simulink model "h"  (R2020a)
settings: Solver=FixedStepAuto  StartTime=0.0  StopTime=10.0  FixedStep=1e-3  RelTol=1e-3  EnableMultiTasking=on
undefined symbols (not defined in the file): D10, D11, D2, D4, D5, D6, D8, PTA0, PTA2, PTB23, PTB9, PTC2, PTD0, PTD2
libraries: frdmk64flib x7
settings Model: ExtModeTrigDuration=5  Creator=qasim  LastModifiedBy=hinda
settings OptimizationCC: EnhancedBackFolding=on  PassReuseOutputArgsAs=Individual arguments  ZeroExternalMemoryAtStartup=off  ZeroInternalMemoryAtStartup=off  MaxStackSize=64  OptimizeBlockOrder=speed  DifferentSizesBufferReuse=on  OptimizationCustomize=off  EfficientTunableParamExpr=on
settings DebuggingCC: ParameterTunabilityLossMsg=error
settings HardwareCC: ProdBitPerPointer=32  ProdBitPerSizeT=32  ProdBitPerPtrDiffT=32  ProdLargestAtomicInteger=Long  ProdLargestAtomicFloat=Double  ProdWordSize=32  ProdHWDeviceType=ARM Compatible->ARM Cortex
settings SFSimCC: MATLABDynamicMemAlloc=off
settings RTWCC: SystemTargetFile=ert.tlc  HardwareBoard=NXP FRDM-K64F  TemplateMakefile=ert_default_tmf  Toolchain=GNU Tools for ARM Embedded Processors
settings CodeAppCC: ForceParamTrailComments=on  IgnoreCustomStorageClasses=off  OperatorAnnotations=on  SimulinkDataObjDesc=on  SFDataObjDesc=on  InsertBlockDesc=on

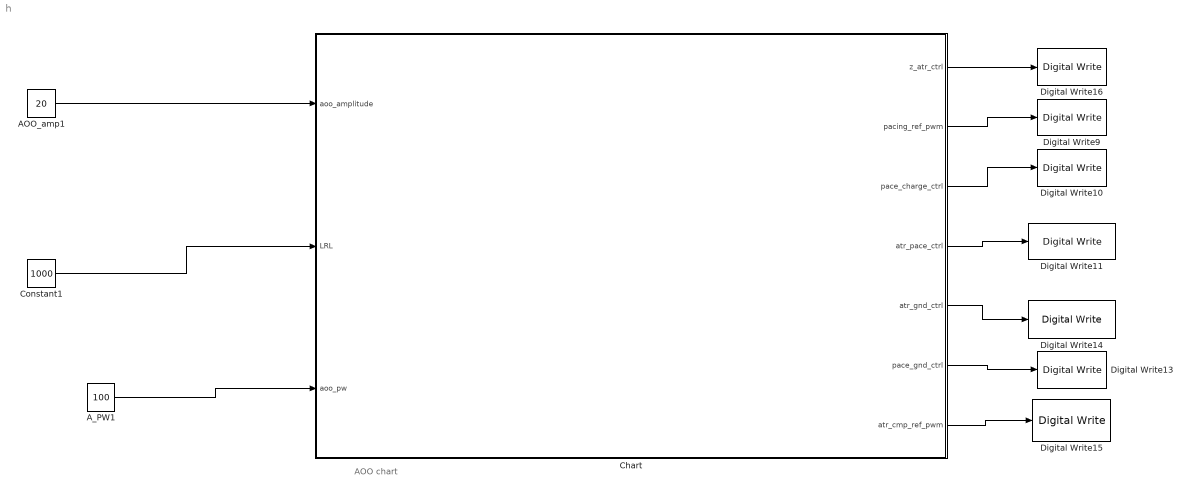
== system h ==
  note: AOO chart
  AOO_amp1 : Constant  Value=20
  A_PW1 : Constant  Value=100
  Chart : Stateflow chart  TreatAsAtomicUnit=on
  Constant1 : Constant  Value=1000
  Digital Write10 : frdmk64flib/Digital Write  Whichpin=PTB9 (D2)
  Digital Write11 : frdmk64flib/Digital Write  Whichpin=PTA0 (D8)
  Digital Write13 : frdmk64flib/Digital Write  Whichpin=PTD0 (D10)
  Digital Write14 : frdmk64flib/Digital Write  Whichpin=PTD2 (D11)
  Digital Write15 : frdmk64flib/Digital Write  Whichpin=PTC2 (D6)
  Digital Write16 : frdmk64flib/Digital Write  Whichpin=PTB23 (D4)
  Digital Write9 : frdmk64flib/Digital Write  Whichpin=PTA2 (D5)
  wires:
  Chart/7(atr_cmp_ref_pwm) -> Digital Write15/1
  Chart/6(pace_gnd_ctrl) -> Digital Write13/1
  Chart/5(atr_gnd_ctrl) -> Digital Write14/1
  Chart/4(atr_pace_ctrl) -> Digital Write11/1
  Chart/3(pace_charge_ctrl) -> Digital Write10/1
  Chart/2(pacing_ref_pwm) -> Digital Write9/1
  Chart/1(z_atr_ctrl) -> Digital Write16/1
  AOO_amp1/1 -> Chart/1(aoo_amplitude)
  Constant1/1 -> Chart/2(LRL)
  A_PW1/1 -> Chart/3(aoo_pw)

== stateflow chart h/Chart ==
  state charging
    entry:
    %charging C22
    %discharging C21
    atr_pace_ctrl = 0; %do not want c22 to discharge
    pacing_ref_pwm = aoo_amplitude; %send in signal
    pace_charge_ctrl = 1;
    pace_gnd_ctrl = 0; %discharges C21
    atr_gnd_ctrl = 1; %1 when discharging through atrium
    atr_cmp_ref_pwm = 80; %send in threshold signal, if heart is less then we will send signal, idk
    %average threshold amplitude is 80
    z_atr_ctrl = 0; %connects impedance circuit to atrium ring electrode output is at z_signal pin
  state pacing
    entry:
    %charging C21
    %discharging C22
    atr_gnd_ctrl = 0;
    atr_pace_ctrl = 1;
    z_atr_ctrl = 0;
    pace_charge_ctrl = 0;
    pace_gnd_ctrl = 1;
    atr_gnd_ctrl = 0;
    pacing_ref_pwm = aoo_amplitude;
  (default) -> charging
  charging -> pacing : [after(aoo_pw, msec)]
  pacing -> charging : [after(LRL - aoo_pw, msec)]
  data: aoo_amplitude input; LRL input; aoo_pw input; z_atr_ctrl output; pacing_ref_pwm output; pace_charge_ctrl output; atr_pace_ctrl output; atr_gnd_ctrl output; pace_gnd_ctrl output; atr_cmp_ref_pwm output
